simulink model "Practica4PID de la práctica 2 modificado"  (R2014b)
settings: Solver=ode45  StartTime=0.0  StopTime=100  RelTol=1e-3
libraries: simulink x1
settings Model: Creator=usuario_local  LastModifiedBy=usuario_local

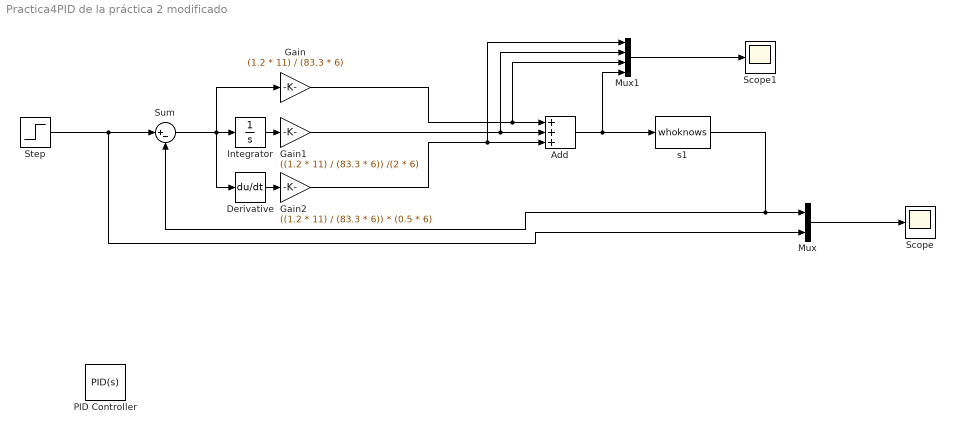
== system Practica4PID de la práctica 2 modificado ==
  Add : Sum  Inputs=+++
  Derivative : Derivative
  Gain : Gain  Gain=(1.2 * 11) / (83.3 * 6)
  Gain1 : Gain  Gain=((1.2 * 11) / (83.3 * 6)) /(2 * 6)
  Gain2 : Gain  Gain=((1.2 * 11) / (83.3 * 6)) * (0.5 * 6)
  Integrator : Integrator
  Mux : Mux  Inputs=2
  Mux1 : Mux
  PID Controller : simulink/Continuous/PID Controller  Controller=PID  TimeDomain=Continuous-time  SampleTime=-1  IntegratorMethod=Forward Euler  FilterMethod=Forward Euler  Form=Parallel  P=(1.2 * 11) / (83.3 * 6)  I=((1.2 * 11) / (83.3 * 6)) /(2 * 6)  D=((1.2 * 11) / (83.3 * 6)) * (0.5 * 6)  N=100  InitialConditionSource=internal  InitialConditionForIntegrator=0  InitialConditionForFilter=0  ExternalReset=none  LimitOutput=off  UpperSaturationLimit=inf  LowerSaturationLimit=-inf  LinearizeAsGain=on  AntiWindupMode=none  Kb=1  TrackingMode=off  Kt=1  PParamMin=[]  PParamMax=[]  IParamMin=[]  IParamMax=[]  DParamMin=[]  DParamMax=[]  NParamMin=[]  NParamMax=[]  KbParamMin=[]  KbParamMax=[]  KtParamMin=[]  KtParamMax=[]  POutMin=[]  POutMax=[]  IOutMin=[]  IOutMax=[]  DOutMin=[]  DOutMax=[]  NOutMin=[]  NOutMax=[]  KbOutMin=[]  KbOutMax=[]  KtOutMin=[]  KtOutMax=[]  IntegratorOutMin=[]  IntegratorOutMax=[]  FilterOutMin=[]  FilterOutMax=[]  SumOutMin=[]  SumOutMax=[]  SumI1OutMin=[]  SumI1OutMax=[]  SumI2OutMin=[]  SumI2OutMax=[]  SumI3OutMin=[]  SumI3OutMax=[]  SumDOutMin=[]  SumDOutMax=[]  SaturationOutMin=[]  SaturationOutMax=[]  IntegratorContinuousStateAttributes=''  IntegratorStateMustResolveToSignalObject=off  IntegratorRTWStateStorageClass=Auto  FilterContinuousStateAttributes=''  FilterStateMustResolveToSignalObject=off  FilterRTWStateStorageClass=Auto  DifferentiatorICPrevScaledInput=0  DifferentiatorOutMin=[]  DifferentiatorOutMax=[]  UseFilter=on
  Scope : Scope
      settings: YMin=-0.2  YMax=1.2
  Scope1 : Scope
  Step : Step  Time=0  SampleTime=0
  Sum : Sum  Inputs=|+-
  s1 : M-S-Function  FunctionName=whoknows  Parameters=L, P1, P2, T, R  mask{L=6, P1=0, P2=3, T=1, R=0}
      mask prompts: L "Laboratorio"; P1 "Primer digito del Puesto"; P2 "Segundo digito del Puesto"; T "Tipo de Planta"; R "Ruido"
      mask Display: disp('Sistema')
  wires:
  s1/1 -> Sum/2, Mux/1
  Step/1 -> Mux/2, Sum/1
  Mux/1 -> Scope/1
  Sum/1 -> Gain/1, Integrator/1, Derivative/1
  Integrator/1 -> Gain1/1
  Derivative/1 -> Gain2/1
  Gain1/1 -> Mux1/2, Add/2
  Add/1 -> Mux1/4, s1/1
  Gain/1 -> Mux1/3, Add/1
  Gain2/1 -> Mux1/1, Add/3
  Mux1/1 -> Scope1/1
